simulink model "mrefrobotarm_modified_previous_y_previous_u_previous_ref"  (R2018b)
settings: Solver=FixedStepAuto  StartTime=0.0  StopTime=10  RelTol=1e-3  AbsTol=1e-6
undefined symbols (not defined in the file or in its folder): options, sfunxy2
libraries: neural x949, simulink x1
(part 20 of 31)

== system mrefrobotarm_modified_previous_y_previous_u_previous_ref/const_51traces_30x30/Layer 3/Delays 1 ==
  "p{3}" : Inport  PortDimensions=30
      mask Display: e = 0.06;c1 = [120 230 180]/255;c2 = ([120 230 180]+0)/(256+128);c3 = ([120 230 180]+128)/(256+128);patch([0 1 1 0],[0 0 1 1],c1);patch([0 1 1 1-e 1-e 0+e],[0 0 1 1-e 0+e 0+e],c2);patch([0 0 1 1-e 0+e 0+e],[0 1 1 1-e 1-e 0+e],c3);plot([0 1 1 0 0],[0 0 1 1 0]);
  mux : Mux  Inputs=1
      mask Display: e = 0.06;c1 = [120 150 230]/255;c2 = ([120 150 230]+0)/383;c3 = ([120 150 230]+128)/383;patch([0 1 1 0],[0 0 1 1],c1);patch([0 1 1 1-e 1-e 0+e],[0 0 1 1-e 0+e 0+e],c2);patch([0 0 1 1-e 0+e 0+e],[0 1 1 1-e 1-e 0+e],c3);plot([0 1 1 0 0],[0 0 1 1 0]);disp('Mux')
  "pd{3,2}" : Outport
      mask Display: e = 0.06;c1 = [120 230 180]/255;c2 = ([120 230 180]+0)/(256+128);c3 = ([120 230 180]+128)/(256+128);patch([0 1 1 0],[0 0 1 1],c1);patch([0 1 1 1-e 1-e 0+e],[0 0 1 1-e 0+e 0+e],c2);patch([0 0 1 1-e 0+e 0+e],[0 1 1 1-e 1-e 0+e],c3);plot([0 1 1 0 0],[0 0 1 1 0]);
  wires:
  "p{3}"/1 -> mux/1
  mux/1 -> "pd{3,2}"/1

== system mrefrobotarm_modified_previous_y_previous_u_previous_ref/const_51traces_30x30/Layer 3/LW{3,2} ==
  "ad{3,2}" : Inport  PortDimensions=30
      mask Display: e = 0.06;c1 = [120 230 180]/255;c2 = ([120 230 180]+0)/(256+128);c3 = ([120 230 180]+128)/(256+128);patch([0 1 1 0],[0 0 1 1],c1);patch([0 1 1 1-e 1-e 0+e],[0 0 1 1-e 0+e 0+e],c2);patch([0 0 1 1-e 0+e 0+e],[0 1 1 1-e 1-e 0+e],c3);plot([0 1 1 0 0],[0 0 1 1 0]);
  "IW{3,2}(1,:)'" : Constant  Value=[-0.2502783511027504292911771699436940252780914306640625;-0.2022822921586699129736786062494502402842044830322265625;0.0138263679365888091099545675888293772004544734954833984375;0.003587340880345798489747810577910058782435953617095947265625;-0.36388265228327398848051643653889186680316925048828125;-0.528173021295331057700650490005500614643096923828125;-0.01174620981264731627013997439235026831738650798797607421875;-0.026166126793346781986837612521412665955722332000732421875;-0.10153833914323888432118536684356513433158397674560546875;0.393125498371538928399360202092793770134449005126953125;0.2121816067702506358738645531047950498759746551513671875;-0.388988456055229026020469973445869982242584228515625;-0.586377978734434979202205795445479452610015869140625;-0.07580851317005264655701779474838986061513423919677734375;0.213741694444092578120120151652372442185878753662109375;0.045896444923178493502380348445512936450541019439697265625;-0.02022614202283436191098786594011471606791019439697265625;-0.66790357501746477897341947027598507702350616455078125;0.62219683659344304782479184723342768847942352294921875;0.038338041364909265784621794637132552452385425567626953125;-0.038180044731395600121626188183654448948800563812255859375;-0.370502103719563991024443794231046922504901885986328125;-0.41852454079916590057308667383040301501750946044921875;-0.22243507530401185334767433232627809047698974609375;0.74163075209700146661617736754124052822589874267578125;0.34077911775747171674311175593174993991851806640625;-0.225161957342794372127769975122646428644657135009765625;0.4331423101356366434089295580633915960788726806640625;-0.06801259193762883292766474596646730788052082061767578125;0.01793271831975769281530830312476609833538532257080078125]
      mask Display: e = 0.06;c1 = [120 150 230]/255;c2 = ([120 150 230]+0)/383;c3 = ([120 150 230]+128)/383;patch([0 1 1 0],[0 0 1 1],c1);patch([0 1 1 1-e 1-e 0+e],[0 0 1 1-e 0+e 0+e],c2);patch([0 0 1 1-e 0+e 0+e],[0 1 1 1-e 1-e 0+e],c3);plot([0 1 1 0 0],[0 0 1 1 0]);disp('weights');
  Mux : Mux  Inputs=1
      mask Display: e = 0.06;c1 = [120 150 230]/255;c2 = ([120 150 230]+0)/383;c3 = ([120 150 230]+128)/383;patch([0 1 1 0],[0 0 1 1],c1);patch([0 1 1 1-e 1-e 0+e],[0 0 1 1-e 0+e 0+e],c2);patch([0 0 1 1-e 0+e 0+e],[0 1 1 1-e 1-e 0+e],c3);plot([0 1 1 0 0],[0 0 1 1 0]);disp('Mux');
  dotprod1 : neural/Weight Functions/dotprod
  "lz{3,2}" : Outport
      mask Display: e = 0.06;c1 = [120 230 180]/255;c2 = ([120 230 180]+0)/(256+128);c3 = ([120 230 180]+128)/(256+128);patch([0 1 1 0],[0 0 1 1],c1);patch([0 1 1 1-e 1-e 0+e],[0 0 1 1-e 0+e 0+e],c2);patch([0 0 1 1-e 0+e 0+e],[0 1 1 1-e 1-e 0+e],c3);plot([0 1 1 0 0],[0 0 1 1 0]);
  wires:
  "IW{3,2}(1,:)'"/1 -> dotprod1/1
  "ad{3,2}"/1 -> dotprod1/2
  dotprod1/1 -> Mux/1
  Mux/1 -> "lz{3,2}"/1

== system mrefrobotarm_modified_previous_y_previous_u_previous_ref/const_51traces_30x30_σ_0.0001/Layer 1/Delays 1 ==
  "p{1}" : Inport  PortDimensions=10
      mask Display: e = 0.06;c1 = [120 230 180]/255;c2 = ([120 230 180]+0)/(256+128);c3 = ([120 230 180]+128)/(256+128);patch([0 1 1 0],[0 0 1 1],c1);patch([0 1 1 1-e 1-e 0+e],[0 0 1 1-e 0+e 0+e],c2);patch([0 0 1 1-e 0+e 0+e],[0 1 1 1-e 1-e 0+e],c3);plot([0 1 1 0 0],[0 0 1 1 0]);
  mux : Mux  Inputs=1
      mask Display: e = 0.06;c1 = [120 150 230]/255;c2 = ([120 150 230]+0)/383;c3 = ([120 150 230]+128)/383;patch([0 1 1 0],[0 0 1 1],c1);patch([0 1 1 1-e 1-e 0+e],[0 0 1 1-e 0+e 0+e],c2);patch([0 0 1 1-e 0+e 0+e],[0 1 1 1-e 1-e 0+e],c3);plot([0 1 1 0 0],[0 0 1 1 0]);disp('Mux')
  "pd{1,1}" : Outport
      mask Display: e = 0.06;c1 = [120 230 180]/255;c2 = ([120 230 180]+0)/(256+128);c3 = ([120 230 180]+128)/(256+128);patch([0 1 1 0],[0 0 1 1],c1);patch([0 1 1 1-e 1-e 0+e],[0 0 1 1-e 0+e 0+e],c2);patch([0 0 1 1-e 0+e 0+e],[0 1 1 1-e 1-e 0+e],c3);plot([0 1 1 0 0],[0 0 1 1 0]);
  wires:
  "p{1}"/1 -> mux/1
  mux/1 -> "pd{1,1}"/1

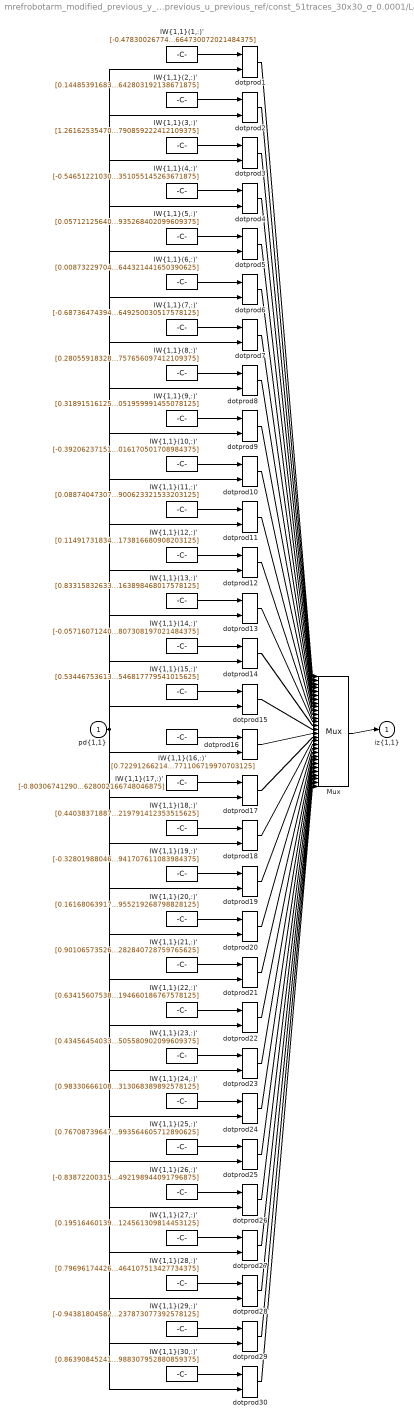
== system mrefrobotarm_modified_previous_y_previous_u_previous_ref/const_51traces_30x30_σ_0.0001/Layer 1/IW{1,1} ==
  "pd{1,1}" : Inport  PortDimensions=10
      mask Display: e = 0.06;c1 = [120 230 180]/255;c2 = ([120 230 180]+0)/(256+128);c3 = ([120 230 180]+128)/(256+128);patch([0 1 1 0],[0 0 1 1],c1);patch([0 1 1 1-e 1-e 0+e],[0 0 1 1-e 0+e 0+e],c2);patch([0 0 1 1-e 0+e 0+e],[0 1 1 1-e 1-e 0+e],c3);plot([0 1 1 0 0],[0 0 1 1 0]);
  "IW{1,1}(1,:)'" : Constant  Value=[-0.4783002677481109632395828157314099371433258056640625;0.225797734006052908117823108113952912390232086181640625;0.0619071299893831639149510692732292227447032928466796875;-0.1305707129982882352958739602399873547255992889404296875;-0.1582316002593976700385525191450142301619052886962890625;0.62738299735823266356504745999700389802455902099609375;-0.07823999424344928177443847516769892536103725433349609375;0.54086962858432408030040505764191038906574249267578125;-1.2308960090184422053738444446935318410396575927734375;-1.1047765761629493308504379456280730664730072021484375]
      mask Display: e = 0.06;c1 = [120 150 230]/255;c2 = ([120 150 230]+0)/383;c3 = ([120 150 230]+128)/383;patch([0 1 1 0],[0 0 1 1],c1);patch([0 1 1 1-e 1-e 0+e],[0 0 1 1-e 0+e 0+e],c2);patch([0 0 1 1-e 0+e 0+e],[0 1 1 1-e 1-e 0+e],c3);plot([0 1 1 0 0],[0 0 1 1 0]);disp('Weights');
  "IW{1,1}(10,:)'" : Constant  Value=[-0.3920623715152447008591707344749011099338531494140625;0.4455119743228426187897639465518295764923095703125;-0.50890894597172720015265667825588025152683258056640625;-1.1274611079542211644621829691459424793720245361328125;-0.494185029516691687323515225216397084295749664306640625;-1.047212236780080463205422347527928650379180908203125;0.39718211885327991961247562358039431273937225341796875;-0.320274894371712137708385625955997966229915618896484375;0.414358439491528895981531377401552163064479827880859375;0.22633357086114302969548361943452619016170501708984375]
      mask Display: e = 0.06;c1 = [120 150 230]/255;c2 = ([120 150 230]+0)/383;c3 = ([120 150 230]+128)/383;patch([0 1 1 0],[0 0 1 1],c1);patch([0 1 1 1-e 1-e 0+e],[0 0 1 1-e 0+e 0+e],c2);patch([0 0 1 1-e 0+e 0+e],[0 1 1 1-e 1-e 0+e],c3);plot([0 1 1 0 0],[0 0 1 1 0]);disp('Weights');
  "IW{1,1}(11,:)'" : Constant  Value=[0.088740473073715520069271178726921789348125457763671875;-0.40773181172127148652606365430983714759349822998046875;0.448640590673554273681844506427296437323093414306640625;-0.9821907998595731381641371626756154000759124755859375;0.28046741465791391600959059360320679843425750732421875;-0.406265214136352914575667227836675010621547698974609375;1.257667551464848987308187133749015629291534423828125;0.24046834669643291082508085310109890997409820556640625;-0.899880726331652613936284978990443050861358642578125;-0.73835995629352890734509173853439278900623321533203125]
      mask Display: e = 0.06;c1 = [120 150 230]/255;c2 = ([120 150 230]+0)/383;c3 = ([120 150 230]+128)/383;patch([0 1 1 0],[0 0 1 1],c1);patch([0 1 1 1-e 1-e 0+e],[0 0 1 1-e 0+e 0+e],c2);patch([0 0 1 1-e 0+e 0+e],[0 1 1 1-e 1-e 0+e],c3);plot([0 1 1 0 0],[0 0 1 1 0]);disp('Weights');
  "IW{1,1}(12,:)'" : Constant  Value=[0.11491731834755421204352643371748854406177997589111328125;-0.47397265770109109350727294440730474889278411865234375;-0.98649203488940007122920405890909023582935333251953125;-0.10177533120774563679677982008797698654234409332275390625;0.592857103007061514432507465244270861148834228515625;0.61221377160847112453012641708482988178730010986328125;-0.9147675167478868107906464501866139471530914306640625;0.12131503446015258484980137154707335866987705230712890625;0.01531316669493529812606791296047958894632756710052490234375;-0.85040691633730614018560345357400365173816680908203125]
      mask Display: e = 0.06;c1 = [120 150 230]/255;c2 = ([120 150 230]+0)/383;c3 = ([120 150 230]+128)/383;patch([0 1 1 0],[0 0 1 1],c1);patch([0 1 1 1-e 1-e 0+e],[0 0 1 1-e 0+e 0+e],c2);patch([0 0 1 1-e 0+e 0+e],[0 1 1 1-e 1-e 0+e],c3);plot([0 1 1 0 0],[0 0 1 1 0]);disp('Weights');
  "IW{1,1}(13,:)'" : Constant  Value=[0.83315832633779984828237274996354244649410247802734375;-0.84813453396239768533604319600271992385387420654296875;0.6587976302083091706407458332250826060771942138671875;0.0287179678210311671582299908322966075502336025238037109375;-0.66940695375002257083707490892265923321247100830078125;0.9950289953187729796724170228117145597934722900390625;0.538080127258940610346371613559313118457794189453125;-0.101113619609701999024764518253505229949951171875;0.01249256520135438690288776086845246027223765850067138671875;0.397809174836881773718033628028933890163898468017578125]
      mask Display: e = 0.06;c1 = [120 150 230]/255;c2 = ([120 150 230]+0)/383;c3 = ([120 150 230]+128)/383;patch([0 1 1 0],[0 0 1 1],c1);patch([0 1 1 1-e 1-e 0+e],[0 0 1 1-e 0+e 0+e],c2);patch([0 0 1 1-e 0+e 0+e],[0 1 1 1-e 1-e 0+e],c3);plot([0 1 1 0 0],[0 0 1 1 0]);disp('Weights');
  "IW{1,1}(14,:)'" : Constant  Value=[-0.057160712406484660841332612335463636554777622222900390625;-1.089057439374407909582487263833172619342803955078125;0.730197751881231482684597722254693508148193359375;-0.403136403292930378672309643661719746887683868408203125;-0.91149829502635271172295006181229837238788604736328125;1.398563629187665302566756508895196020603179931640625;0.425389740709256003459159956037183292210102081298828125;0.1041973624263145270507635586909600533545017242431640625;-0.290427050222273663848682190291583538055419921875;0.0704235764473631620230520411496399901807308197021484375]
      mask Display: e = 0.06;c1 = [120 150 230]/255;c2 = ([120 150 230]+0)/383;c3 = ([120 150 230]+128)/383;patch([0 1 1 0],[0 0 1 1],c1);patch([0 1 1 1-e 1-e 0+e],[0 0 1 1-e 0+e 0+e],c2);patch([0 0 1 1-e 0+e 0+e],[0 1 1 1-e 1-e 0+e],c3);plot([0 1 1 0 0],[0 0 1 1 0]);disp('Weights');
  "IW{1,1}(15,:)'" : Constant  Value=[0.53446753613595354703846851407433860003948211669921875;-0.351963242971691625537999925654730759561061859130859375;0.80470610943757991950775476652779616415500640869140625;0.334929837316443490546902239657356403768062591552734375;-0.0243479361781237697848201406713997130282223224639892578125;-0.90212937554959893304840079508721828460693359375;-0.679774148371051989414581839810125529766082763671875;0.3560781837998734378203380401828326284885406494140625;0.99704236367271603658224421451450325548648834228515625;-0.364711068944728877827543556122691370546817779541015625]
      mask Display: e = 0.06;c1 = [120 150 230]/255;c2 = ([120 150 230]+0)/383;c3 = ([120 150 230]+128)/383;patch([0 1 1 0],[0 0 1 1],c1);patch([0 1 1 1-e 1-e 0+e],[0 0 1 1-e 0+e 0+e],c2);patch([0 0 1 1-e 0+e 0+e],[0 1 1 1-e 1-e 0+e],c3);plot([0 1 1 0 0],[0 0 1 1 0]);disp('Weights');
  "IW{1,1}(16,:)'" : Constant  Value=[0.72291266214445482063410963746719062328338623046875;-1.193145409928211275740750352269969880580902099609375;-0.5937483283746562978677729915943928062915802001953125;0.867343354951155109944238574826158583164215087890625;-0.2133625292175349574819165354711003601551055908203125;-0.68845640268906571623830359385465271770954132080078125;0.145533828666085884862013699603267014026641845703125;-0.317244368543982135921766030151047743856906890869140625;0.38202589330718428328736990806646645069122314453125;0.07742204349810129226927557510862243361771106719970703125]
      mask Display: e = 0.06;c1 = [120 150 230]/255;c2 = ([120 150 230]+0)/383;c3 = ([120 150 230]+128)/383;patch([0 1 1 0],[0 0 1 1],c1);patch([0 1 1 1-e 1-e 0+e],[0 0 1 1-e 0+e 0+e],c2);patch([0 0 1 1-e 0+e 0+e],[0 1 1 1-e 1-e 0+e],c3);plot([0 1 1 0 0],[0 0 1 1 0]);disp('Weights');
  "IW{1,1}(17,:)'" : Constant  Value=[-0.8030674129022485896456373666296713054180145263671875;-0.166538028663690329533864087352412752807140350341796875;-0.63407164183701769655243651868659071624279022216796875;-0.62438168176794395236584023223258554935455322265625;-0.308951728432432959348119538844912312924861907958984375;1.04665400285656406964562847861088812351226806640625;0.402742716949034906814830492294277064502239227294921875;-0.3276909436173232048616910105920396745204925537109375;0.1191040517349247485068275409503257833421230316162109375;0.83243052306274289975362989935092628002166748046875]
      mask Display: e = 0.06;c1 = [120 150 230]/255;c2 = ([120 150 230]+0)/383;c3 = ([120 150 230]+128)/383;patch([0 1 1 0],[0 0 1 1],c1);patch([0 1 1 1-e 1-e 0+e],[0 0 1 1-e 0+e 0+e],c2);patch([0 0 1 1-e 0+e 0+e],[0 1 1 1-e 1-e 0+e],c3);plot([0 1 1 0 0],[0 0 1 1 0]);disp('Weights');
  "IW{1,1}(18,:)'" : Constant  Value=[0.44038371887304250673622618705849163234233856201171875;0.3074991266855675586811003086040727794170379638671875;0.9876290774032894237421942307264544069766998291015625;-0.35518165972444781797179302884615026414394378662109375;0.1326469951829168658630209165494306944310665130615234375;0.497482940534406503640951768829836510121822357177734375;0.6336152023166103930407189182005822658538818359375;-0.970452252277989924067469473811797797679901123046875;0.8921723072545972854641149751842021942138671875;-0.00391263466717305975761664882384138763882219791412353515625]
      mask Display: e = 0.06;c1 = [120 150 230]/255;c2 = ([120 150 230]+0)/383;c3 = ([120 150 230]+128)/383;patch([0 1 1 0],[0 0 1 1],c1);patch([0 1 1 1-e 1-e 0+e],[0 0 1 1-e 0+e 0+e],c2);patch([0 0 1 1-e 0+e 0+e],[0 1 1 1-e 1-e 0+e],c3);plot([0 1 1 0 0],[0 0 1 1 0]);disp('Weights');
  "IW{1,1}(19,:)'" : Constant  Value=[-0.32801988046943364452090463601052761077880859375;0.94992233620265287274975207765237428247928619384765625;-0.0931813581971525362046548934813472442328929901123046875;0.624674388295734406284509532270021736621856689453125;0.27953618933790702616448697881423868238925933837890625;0.6345514494240738212482710878248326480388641357421875;0.8951720419239406201228348436416126787662506103515625;-0.136186452371050481513492513840901665389537811279296875;-0.294617872829695037761865705761010758578777313232421875;-0.68270472391063863337734574088244698941707611083984375]
      mask Display: e = 0.06;c1 = [120 150 230]/255;c2 = ([120 150 230]+0)/383;c3 = ([120 150 230]+128)/383;patch([0 1 1 0],[0 0 1 1],c1);patch([0 1 1 1-e 1-e 0+e],[0 0 1 1-e 0+e 0+e],c2);patch([0 0 1 1-e 0+e 0+e],[0 1 1 1-e 1-e 0+e],c3);plot([0 1 1 0 0],[0 0 1 1 0]);disp('Weights');
  "IW{1,1}(2,:)'" : Constant  Value=[0.1448539168319732672873811907265917398035526275634765625;1.0687971129812592341323806977015919983386993408203125;-0.07670068689463342692658187615961651317775249481201171875;0.23471894136307380751560458520543761551380157470703125;-0.62624409602090425064346845829277299344539642333984375;0.7121221149727647858895807075896300375461578369140625;0.356617441452001193713527982254163362085819244384765625;0.947917558304493201859486362081952393054962158203125;-0.8872301437075729158010517494403757154941558837890625;0.419187129032490446434167097322642803192138671875]
      mask Display: e = 0.06;c1 = [120 150 230]/255;c2 = ([120 150 230]+0)/383;c3 = ([120 150 230]+128)/383;patch([0 1 1 0],[0 0 1 1],c1);patch([0 1 1 1-e 1-e 0+e],[0 0 1 1-e 0+e 0+e],c2);patch([0 0 1 1-e 0+e 0+e],[0 1 1 1-e 1-e 0+e],c3);plot([0 1 1 0 0],[0 0 1 1 0]);disp('Weights');
  "IW{1,1}(20,:)'" : Constant  Value=[0.1616806391788585817170798009101417846977710723876953125;-0.46469255130542108656044320014188997447490692138671875;1.163665910473917985967773347510956227779388427734375;0.437474148205290680468948494308278895914554595947265625;-0.571555540938710304743608503486029803752899169921875;-0.758881844319549525579304827260784804821014404296875;-0.197593623437410770282696148569812066853046417236328125;0.028604262162167805316759228162482031621038913726806640625;0.699743138197329361815945958369411528110504150390625;-0.439378349202449058896746691971202380955219268798828125]
      mask Display: e = 0.06;c1 = [120 150 230]/255;c2 = ([120 150 230]+0)/383;c3 = ([120 150 230]+128)/383;patch([0 1 1 0],[0 0 1 1],c1);patch([0 1 1 1-e 1-e 0+e],[0 0 1 1-e 0+e 0+e],c2);patch([0 0 1 1-e 0+e 0+e],[0 1 1 1-e 1-e 0+e],c3);plot([0 1 1 0 0],[0 0 1 1 0]);disp('Weights');
  "IW{1,1}(21,:)'" : Constant  Value=[0.90106573526876143631625382113270461559295654296875;-1.1559173660122323834542612530640326440334320068359375;-0.68957746785386075938362182569107972085475921630859375;-0.2616171785124234983044289037934504449367523193359375;0.466512094123854803573436811348074115812778472900390625;-0.45648647436032663282645671642967499792575836181640625;0.373099822895134825007090739745763130486011505126953125;-0.57044042184486765112438888536416925489902496337890625;0.380723636551317634602042971891933120787143707275390625;0.10507997803709069606359349791091517545282840728759765625]
      mask Display: e = 0.06;c1 = [120 150 230]/255;c2 = ([120 150 230]+0)/383;c3 = ([120 150 230]+128)/383;patch([0 1 1 0],[0 0 1 1],c1);patch([0 1 1 1-e 1-e 0+e],[0 0 1 1-e 0+e 0+e],c2);patch([0 0 1 1-e 0+e 0+e],[0 1 1 1-e 1-e 0+e],c3);plot([0 1 1 0 0],[0 0 1 1 0]);disp('Weights');
  "IW{1,1}(22,:)'" : Constant  Value=[0.63415607538566909351374079051311127841472625732421875;-0.91039462852150798699568667871062643826007843017578125;-0.0074177170721081674142904915925100794993340969085693359375;0.85140437325898787879197016081889159977436065673828125;-0.265936880568247657752323220847756601870059967041015625;0.0164960299259189653586776813654068973846733570098876953125;-1.01287933676323493870086167589761316776275634765625;0.1738081331760349679260713173789554275572299957275390625;0.55736963074007228602368968495284207165241241455078125;-0.73070603044738569042948483911459334194660186767578125]
      mask Display: e = 0.06;c1 = [120 150 230]/255;c2 = ([120 150 230]+0)/383;c3 = ([120 150 230]+128)/383;patch([0 1 1 0],[0 0 1 1],c1);patch([0 1 1 1-e 1-e 0+e],[0 0 1 1-e 0+e 0+e],c2);patch([0 0 1 1-e 0+e 0+e],[0 1 1 1-e 1-e 0+e],c3);plot([0 1 1 0 0],[0 0 1 1 0]);disp('Weights');
  "IW{1,1}(23,:)'" : Constant  Value=[0.434564540335410587346132160746492445468902587890625;-0.0217634792451496909826413883592977072112262248992919921875;-0.5635401919912224055764227159670554101467132568359375;0.60908933933864151111237106306361965835094451904296875;0.6002121822139876439194949853117577731609344482421875;0.162553268374114268102204050592263229191303253173828125;0.8929541354775512029817718939739279448986053466796875;-1.032658901296135578462553894496522843837738037109375;0.369059645141419367941892915041535161435604095458984375;-0.762472416757764559491761247045360505580902099609375]
      mask Display: e = 0.06;c1 = [120 150 230]/255;c2 = ([120 150 230]+0)/383;c3 = ([120 150 230]+128)/383;patch([0 1 1 0],[0 0 1 1],c1);patch([0 1 1 1-e 1-e 0+e],[0 0 1 1-e 0+e 0+e],c2);patch([0 0 1 1-e 0+e 0+e],[0 1 1 1-e 1-e 0+e],c3);plot([0 1 1 0 0],[0 0 1 1 0]);disp('Weights');
  "IW{1,1}(24,:)'" : Constant  Value=[0.98330666108479747311577057189424522221088409423828125;0.1710542382120223969810268727087532170116901397705078125;0.150621297840954737612406688640476204454898834228515625;-0.513279070999530961927348471363075077533721923828125;0.79017623621034738246038386932923458516597747802734375;0.98157763357863869746466889409930445253849029541015625;-0.74215222271081204841181033771135844290256500244140625;0.326746039040374192108373563314671628177165985107421875;0.6894855111388997759291896727518178522586822509765625;0.25865053304279606027904492293600924313068389892578125]
      mask Display: e = 0.06;c1 = [120 150 230]/255;c2 = ([120 150 230]+0)/383;c3 = ([120 150 230]+128)/383;patch([0 1 1 0],[0 0 1 1],c1);patch([0 1 1 1-e 1-e 0+e],[0 0 1 1-e 0+e 0+e],c2);patch([0 0 1 1-e 0+e 0+e],[0 1 1 1-e 1-e 0+e],c3);plot([0 1 1 0 0],[0 0 1 1 0]);disp('Weights');
  "IW{1,1}(25,:)'" : Constant  Value=[0.7670873964721407478606352015049196779727935791015625;0.00772407323657823934037747193315226468257606029510498046875;0.75709149850982282448086380099994130432605743408203125;-0.65260253848545157762117696620407514274120330810546875;-0.69764480443075960192089723932440392673015594482421875;0.9770356314513808371202685520984232425689697265625;-0.3870063887055577023232899591675959527492523193359375;0.470529924556381706768348749392316676676273345947265625;-0.478279958975531716003359861133503727614879608154296875;0.82813915466962451095156438896083272993564605712890625]
      mask Display: e = 0.06;c1 = [120 150 230]/255;c2 = ([120 150 230]+0)/383;c3 = ([120 150 230]+128)/383;patch([0 1 1 0],[0 0 1 1],c1);patch([0 1 1 1-e 1-e 0+e],[0 0 1 1-e 0+e 0+e],c2);patch([0 0 1 1-e 0+e 0+e],[0 1 1 1-e 1-e 0+e],c3);plot([0 1 1 0 0],[0 0 1 1 0]);disp('Weights');
  "IW{1,1}(26,:)'" : Constant  Value=[-0.8387220031557907073960222987807355821132659912109375;0.55629251053957784467485225832206197082996368408203125;0.85783978317718034833916362913441844284534454345703125;0.61381976325923492954217408623662777245044708251953125;-0.3971923701137802797944686972186900675296783447265625;-0.036173563998751233350414935330263688229024410247802734375;0.280098501895951479401247752321069128811359405517578125;0.82366504778413285325910919709713198244571685791015625;-0.920416110493146089055471747997216880321502685546875;-0.224795494922506111645787996167200617492198944091796875]
      mask Display: e = 0.06;c1 = [120 150 230]/255;c2 = ([120 150 230]+0)/383;c3 = ([120 150 230]+128)/383;patch([0 1 1 0],[0 0 1 1],c1);patch([0 1 1 1-e 1-e 0+e],[0 0 1 1-e 0+e 0+e],c2);patch([0 0 1 1-e 0+e 0+e],[0 1 1 1-e 1-e 0+e],c3);plot([0 1 1 0 0],[0 0 1 1 0]);disp('Weights');
  "IW{1,1}(27,:)'" : Constant  Value=[0.19516460139056046596550686444970779120922088623046875;0.66510373616997420231911064547603018581867218017578125;-0.58845460901194746039521987768239341676235198974609375;0.60114580477881618403301899888901971280574798583984375;-0.257561435963020668449274808153859339654445648193359375;-0.69667742499880114248611562288715504109859466552734375;1.1148557291252270129433554757270030677318572998046875;0.25923365714179780194825752914766781032085418701171875;-0.62752283531356989332294915584498085081577301025390625;0.6133797408613237411856289327261038124561309814453125]
      mask Display: e = 0.06;c1 = [120 150 230]/255;c2 = ([120 150 230]+0)/383;c3 = ([120 150 230]+128)/383;patch([0 1 1 0],[0 0 1 1],c1);patch([0 1 1 1-e 1-e 0+e],[0 0 1 1-e 0+e 0+e],c2);patch([0 0 1 1-e 0+e 0+e],[0 1 1 1-e 1-e 0+e],c3);plot([0 1 1 0 0],[0 0 1 1 0]);disp('Weights');
  "IW{1,1}(28,:)'" : Constant  Value=[0.7969617442699326037569562686257995665073394775390625;-0.9337759685667441633682983592734672129154205322265625;-0.300003587658774772961578491958789527416229248046875;-0.442585244194095117631349012299324385821819305419921875;0.550186661350819949944934705854393541812896728515625;-0.372565647011661560394912839910830371081829071044921875;0.71394276252159738493929808100801892578601837158203125;0.86955905743556860532095242888317443430423736572265625;-0.048946729057372469207098930610300158150494098663330078125;0.336153630936558922570611684932373464107513427734375]
      mask Display: e = 0.06;c1 = [120 150 230]/255;c2 = ([120 150 230]+0)/383;c3 = ([120 150 230]+128)/383;patch([0 1 1 0],[0 0 1 1],c1);patch([0 1 1 1-e 1-e 0+e],[0 0 1 1-e 0+e 0+e],c2);patch([0 0 1 1-e 0+e 0+e],[0 1 1 1-e 1-e 0+e],c3);plot([0 1 1 0 0],[0 0 1 1 0]);disp('Weights');
  "IW{1,1}(29,:)'" : Constant  Value=[-0.94381804582056283425828269173507578670978546142578125;0.367179809012225077946567353137652389705181121826171875;1.0862025113337530068946534811402671039104461669921875;-0.87717802767758723536672960108262486755847930908203125;0.28712505417192080159338729572482407093048095703125;0.0035962786625754277446131990103594944230280816555023193359375;-0.280731559761747850867408260455704294145107269287109375;-0.2060156830098024693942448948291712440550327301025390625;0.4320099014266671755279958233586512506008148193359375;-0.79722816985893907304472350006108172237873077392578125]
      mask Display: e = 0.06;c1 = [120 150 230]/255;c2 = ([120 150 230]+0)/383;c3 = ([120 150 230]+128)/383;patch([0 1 1 0],[0 0 1 1],c1);patch([0 1 1 1-e 1-e 0+e],[0 0 1 1-e 0+e 0+e],c2);patch([0 0 1 1-e 0+e 0+e],[0 1 1 1-e 1-e 0+e],c3);plot([0 1 1 0 0],[0 0 1 1 0]);disp('Weights');
  "IW{1,1}(3,:)'" : Constant  Value=[1.261625354703996837457680157967843115329742431640625;-0.827428609105913093202389063662849366664886474609375;-0.351047667779615102379153768197284080088138580322265625;0.4287181311290113594480999381630681455135345458984375;-0.09690495277992121347931941954811918549239635467529296875;-0.1339986688941029180366371065247221849858760833740234375;0.2813056242858122946159937782795168459415435791015625;0.280990867531233146081603990751318633556365966796875;0.164937419584575362119238661762210540473461151123046875;-0.98327685331950609448625755248940549790859222412109375]
      mask Display: e = 0.06;c1 = [120 150 230]/255;c2 = ([120 150 230]+0)/383;c3 = ([120 150 230]+128)/383;patch([0 1 1 0],[0 0 1 1],c1);patch([0 1 1 1-e 1-e 0+e],[0 0 1 1-e 0+e 0+e],c2);patch([0 0 1 1-e 0+e 0+e],[0 1 1 1-e 1-e 0+e],c3);plot([0 1 1 0 0],[0 0 1 1 0]);disp('Weights');
  "IW{1,1}(30,:)'" : Constant  Value=[0.86390845241718938751773748663254082202911376953125;-1.0636457240922096989521605792106129229068756103515625;-0.062427155465566923353559758425035397522151470184326171875;0.82069770503606764844306553641217760741710662841796875;-0.5451539873732531571448589602368883788585662841796875;0.73532791587776424879763226272189058363437652587890625;0.1919423326425182263488267153661581687629222869873046875;-0.50264000536427932974703480795142240822315216064453125;0.166818657897247646371141627241740934550762176513671875;0.451331762701861760600507977869710884988307952880859375]
      mask Display: e = 0.06;c1 = [120 150 230]/255;c2 = ([120 150 230]+0)/383;c3 = ([120 150 230]+128)/383;patch([0 1 1 0],[0 0 1 1],c1);patch([0 1 1 1-e 1-e 0+e],[0 0 1 1-e 0+e 0+e],c2);patch([0 0 1 1-e 0+e 0+e],[0 1 1 1-e 1-e 0+e],c3);plot([0 1 1 0 0],[0 0 1 1 0]);disp('Weights');
  "IW{1,1}(4,:)'" : Constant  Value=[-0.546512210301335787931975573883391916751861572265625;0.63199046925197743806990047232829965651035308837890625;-0.6648501917604938693528993098880164325237274169921875;0.187265210094508083304987167139188386499881744384765625;0.5670338689418528144159381554345600306987762451171875;0.093994908208824778927947818374377675354480743408203125;-0.817114012108385967536605676286853849887847900390625;-0.0121410548173577943764644970769950305111706256866455078125;0.70928789416413529078653255055542103946208953857421875;-0.88448306199756654422117208014242351055145263671875]
      mask Display: e = 0.06;c1 = [120 150 230]/255;c2 = ([120 150 230]+0)/383;c3 = ([120 150 230]+128)/383;patch([0 1 1 0],[0 0 1 1],c1);patch([0 1 1 1-e 1-e 0+e],[0 0 1 1-e 0+e 0+e],c2);patch([0 0 1 1-e 0+e 0+e],[0 1 1 1-e 1-e 0+e],c3);plot([0 1 1 0 0],[0 0 1 1 0]);disp('Weights');
  "IW{1,1}(5,:)'" : Constant  Value=[0.0571212564080200435601142316954792477190494537353515625;0.893655475520423348001486374414525926113128662109375;-0.38787625453751040094374502587015740573406219482421875;1.048588269192153088482655221014283597469329833984375;0.1553736210277976426130663867297698743641376495361328125;-0.459582842374546773900334528661915101110935211181640625;0.3253855578375828283554938025190494954586029052734375;0.0573267400577433250408176945711602456867694854736328125;1.0324609885572015866017636653850786387920379638671875;-0.38266970997354865513528920928365550935268402099609375]
      mask Display: e = 0.06;c1 = [120 150 230]/255;c2 = ([120 150 230]+0)/383;c3 = ([120 150 230]+128)/383;patch([0 1 1 0],[0 0 1 1],c1);patch([0 1 1 1-e 1-e 0+e],[0 0 1 1-e 0+e 0+e],c2);patch([0 0 1 1-e 0+e 0+e],[0 1 1 1-e 1-e 0+e],c3);plot([0 1 1 0 0],[0 0 1 1 0]);disp('Weights');
  "IW{1,1}(6,:)'" : Constant  Value=[0.0087322970414144551742907651714631356298923492431640625;0.70407432440727302225269568225485272705554962158203125;-0.90942850094851224174163917268742807209491729736328125;-1.009443424489020468826083742897026240825653076171875;-0.2181544944626568061085691851985757239162921905517578125;-0.70820009823831731043952686377451755106449127197265625;0.6371367518358150849877574728452600538730621337890625;0.025279539773087007781260382444088463671505451202392578125;0.09679086062483378827270286137718358077108860015869140625;0.46035452825426370626615835135453380644321441650390625]
      mask Display: e = 0.06;c1 = [120 150 230]/255;c2 = ([120 150 230]+0)/383;c3 = ([120 150 230]+128)/383;patch([0 1 1 0],[0 0 1 1],c1);patch([0 1 1 1-e 1-e 0+e],[0 0 1 1-e 0+e 0+e],c2);patch([0 0 1 1-e 0+e 0+e],[0 1 1 1-e 1-e 0+e],c3);plot([0 1 1 0 0],[0 0 1 1 0]);disp('Weights');
  "IW{1,1}(7,:)'" : Constant  Value=[-0.6873647439410455195485383228515274822711944580078125;-0.404620549455107558767252839970751665532588958740234375;-0.50116779611188022602874525546212680637836456298828125;0.11080082968676792376516715421530534513294696807861328125;0.73974873833491894270508737463387660682201385498046875;-0.28577067616393370119709516075090505182743072509765625;0.2330543705783859886881970169270061887800693511962890625;0.96735425271560948612403763036127202212810516357421875;-0.2195245278103102049005457274688524194061756134033203125;-0.59568704784472448210408401791937649250030517578125]
      mask Display: e = 0.06;c1 = [120 150 230]/255;c2 = ([120 150 230]+0)/383;c3 = ([120 150 230]+128)/383;patch([0 1 1 0],[0 0 1 1],c1);patch([0 1 1 1-e 1-e 0+e],[0 0 1 1-e 0+e 0+e],c2);patch([0 0 1 1-e 0+e 0+e],[0 1 1 1-e 1-e 0+e],c3);plot([0 1 1 0 0],[0 0 1 1 0]);disp('Weights');
  "IW{1,1}(8,:)'" : Constant  Value=[0.280559183288091096297733884057379327714443206787109375;-0.77389112175549901184723466940340586006641387939453125;0.391322292075829469837344731786288321018218994140625;-0.333097563073307123548971730997436679899692535400390625;0.178709967830229465857172499454463832080364227294921875;0.97402746195749745350411785693722777068614959716796875;0.026218224234564831143234897581351106055080890655517578125;0.93172243425795875371164811440394259989261627197265625;-0.7614610886790895705189541331492364406585693359375;-0.4920663684245933922056792653165757656097412109375]
      mask Display: e = 0.06;c1 = [120 150 230]/255;c2 = ([120 150 230]+0)/383;c3 = ([120 150 230]+128)/383;patch([0 1 1 0],[0 0 1 1],c1);patch([0 1 1 1-e 1-e 0+e],[0 0 1 1-e 0+e 0+e],c2);patch([0 0 1 1-e 0+e 0+e],[0 1 1 1-e 1-e 0+e],c3);plot([0 1 1 0 0],[0 0 1 1 0]);disp('Weights');
  "IW{1,1}(9,:)'" : Constant  Value=[0.31891516125266805570248607182293199002742767333984375;-0.9590055009861366830392626070533879101276397705078125;0.73873827762571131483326780653442256152629852294921875;0.10576007099043328862908452947522164322435855865478515625;0.46696443698258904841935645890771411359310150146484375;0.867518533528885082972692543989978730678558349609375;0.61804139673547997535507647626218385994434356689453125;0.5114111196921566904194378366810269653797149658203125;0.00631983919589989250054085090368971577845513820648193359375;-0.5902014341754686643781724342261441051959991455078125]
      mask Display: e = 0.06;c1 = [120 150 230]/255;c2 = ([120 150 230]+0)/383;c3 = ([120 150 230]+128)/383;patch([0 1 1 0],[0 0 1 1],c1);patch([0 1 1 1-e 1-e 0+e],[0 0 1 1-e 0+e 0+e],c2);patch([0 0 1 1-e 0+e 0+e],[0 1 1 1-e 1-e 0+e],c3);plot([0 1 1 0 0],[0 0 1 1 0]);disp('Weights');
  Mux : Mux  Inputs=30
      mask Display: e = 0.06;c1 = [120 150 230]/255;c2 = ([120 150 230]+0)/383;c3 = ([120 150 230]+128)/383;patch([0 1 1 0],[0 0 1 1],c1);patch([0 1 1 1-e 1-e 0+e],[0 0 1 1-e 0+e 0+e],c2);patch([0 0 1 1-e 0+e 0+e],[0 1 1 1-e 1-e 0+e],c3);plot([0 1 1 0 0],[0 0 1 1 0]);disp('Mux');
  dotprod{1..30} (30 alike) : neural/Weight Functions/dotprod
  "iz{1,1}" : Outport
      mask Display: e = 0.06;c1 = [120 230 180]/255;c2 = ([120 230 180]+0)/(256+128);c3 = ([120 230 180]+128)/(256+128);patch([0 1 1 0],[0 0 1 1],c1);patch([0 1 1 1-e 1-e 0+e],[0 0 1 1-e 0+e 0+e],c2);patch([0 0 1 1-e 0+e 0+e],[0 1 1 1-e 1-e 0+e],c3);plot([0 1 1 0 0],[0 0 1 1 0]);
  wires:
  "IW{1,1}(1,:)'"/1 -> dotprod1/1
  "pd{1,1}"/1 -> dotprod1/2, dotprod2/2, dotprod3/2, dotprod4/2, dotprod5/2, dotprod6/2, dotprod7/2, dotprod8/2, dotprod9/2, dotprod10/2, dotprod11/2, dotprod12/2, dotprod13/2, dotprod14/2, dotprod15/2, dotprod16/2, dotprod17/2, dotprod18/2, dotprod19/2, dotprod20/2, dotprod21/2, dotprod22/2, dotprod23/2, dotprod24/2, dotprod25/2, dotprod26/2, dotprod27/2, dotprod28/2, dotprod29/2, dotprod30/2
  dotprod1/1 -> Mux/1
  "IW{1,1}(2,:)'"/1 -> dotprod2/1
  dotprod2/1 -> Mux/2
  "IW{1,1}(3,:)'"/1 -> dotprod3/1
  dotprod3/1 -> Mux/3
  "IW{1,1}(4,:)'"/1 -> dotprod4/1
  dotprod4/1 -> Mux/4
  "IW{1,1}(5,:)'"/1 -> dotprod5/1
  dotprod5/1 -> Mux/5
  "IW{1,1}(6,:)'"/1 -> dotprod6/1
  dotprod6/1 -> Mux/6
  "IW{1,1}(7,:)'"/1 -> dotprod7/1
  dotprod7/1 -> Mux/7
  "IW{1,1}(8,:)'"/1 -> dotprod8/1
  dotprod8/1 -> Mux/8
  "IW{1,1}(9,:)'"/1 -> dotprod9/1
  dotprod9/1 -> Mux/9
  "IW{1,1}(10,:)'"/1 -> dotprod10/1
  dotprod10/1 -> Mux/10
  "IW{1,1}(11,:)'"/1 -> dotprod11/1
  dotprod11/1 -> Mux/11
  "IW{1,1}(12,:)'"/1 -> dotprod12/1
  dotprod12/1 -> Mux/12
  "IW{1,1}(13,:)'"/1 -> dotprod13/1
  dotprod13/1 -> Mux/13
  "IW{1,1}(14,:)'"/1 -> dotprod14/1
  dotprod14/1 -> Mux/14
  "IW{1,1}(15,:)'"/1 -> dotprod15/1
  dotprod15/1 -> Mux/15
  "IW{1,1}(16,:)'"/1 -> dotprod16/1
  dotprod16/1 -> Mux/16
  "IW{1,1}(17,:)'"/1 -> dotprod17/1
  dotprod17/1 -> Mux/17
  "IW{1,1}(18,:)'"/1 -> dotprod18/1
  dotprod18/1 -> Mux/18
  "IW{1,1}(19,:)'"/1 -> dotprod19/1
  dotprod19/1 -> Mux/19
  "IW{1,1}(20,:)'"/1 -> dotprod20/1
  dotprod20/1 -> Mux/20
  "IW{1,1}(21,:)'"/1 -> dotprod21/1
  dotprod21/1 -> Mux/21
  "IW{1,1}(22,:)'"/1 -> dotprod22/1
  dotprod22/1 -> Mux/22
  "IW{1,1}(23,:)'"/1 -> dotprod23/1
  dotprod23/1 -> Mux/23
  "IW{1,1}(24,:)'"/1 -> dotprod24/1
  dotprod24/1 -> Mux/24
  "IW{1,1}(25,:)'"/1 -> dotprod25/1
  dotprod25/1 -> Mux/25
  "IW{1,1}(26,:)'"/1 -> dotprod26/1
  dotprod26/1 -> Mux/26
  "IW{1,1}(27,:)'"/1 -> dotprod27/1
  dotprod27/1 -> Mux/27
  "IW{1,1}(28,:)'"/1 -> dotprod28/1
  dotprod28/1 -> Mux/28
  "IW{1,1}(29,:)'"/1 -> dotprod29/1
  dotprod29/1 -> Mux/29
  "IW{1,1}(30,:)'"/1 -> dotprod30/1
  dotprod30/1 -> Mux/30
  Mux/1 -> "iz{1,1}"/1

== system mrefrobotarm_modified_previous_y_previous_u_previous_ref/const_51traces_30x30_σ_0.0001/Layer 2/Delays 1 ==
  "p{2}" : Inport  PortDimensions=30
      mask Display: e = 0.06;c1 = [120 230 180]/255;c2 = ([120 230 180]+0)/(256+128);c3 = ([120 230 180]+128)/(256+128);patch([0 1 1 0],[0 0 1 1],c1);patch([0 1 1 1-e 1-e 0+e],[0 0 1 1-e 0+e 0+e],c2);patch([0 0 1 1-e 0+e 0+e],[0 1 1 1-e 1-e 0+e],c3);plot([0 1 1 0 0],[0 0 1 1 0]);
  mux : Mux  Inputs=1
      mask Display: e = 0.06;c1 = [120 150 230]/255;c2 = ([120 150 230]+0)/383;c3 = ([120 150 230]+128)/383;patch([0 1 1 0],[0 0 1 1],c1);patch([0 1 1 1-e 1-e 0+e],[0 0 1 1-e 0+e 0+e],c2);patch([0 0 1 1-e 0+e 0+e],[0 1 1 1-e 1-e 0+e],c3);plot([0 1 1 0 0],[0 0 1 1 0]);disp('Mux')
  "pd{2,1}" : Outport
      mask Display: e = 0.06;c1 = [120 230 180]/255;c2 = ([120 230 180]+0)/(256+128);c3 = ([120 230 180]+128)/(256+128);patch([0 1 1 0],[0 0 1 1],c1);patch([0 1 1 1-e 1-e 0+e],[0 0 1 1-e 0+e 0+e],c2);patch([0 0 1 1-e 0+e 0+e],[0 1 1 1-e 1-e 0+e],c3);plot([0 1 1 0 0],[0 0 1 1 0]);
  wires:
  "p{2}"/1 -> mux/1
  mux/1 -> "pd{2,1}"/1
